simulink model "n2"  (R2013a)
settings: Solver=ode45  StartTime=0.0  StopTime=time  RelTol=1e-3
values from neighbouring files (symbols this model uses):
  noisePower = 1e3    (= 1000)    [proj.m]
undefined symbols (not defined in the file or in its folder): init, seed
libraries: neural x55, simulink x1
(part 2 of 3)

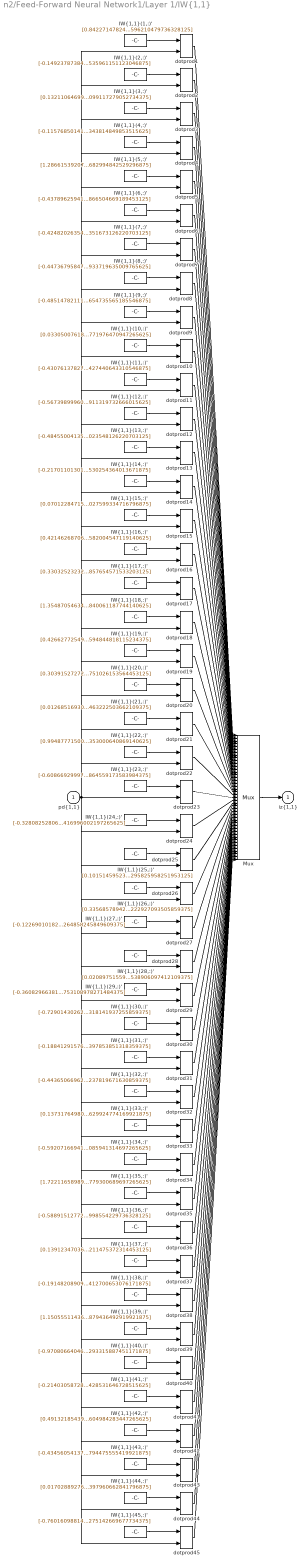
== system n2/Feed-Forward Neural Network1/Layer 1/IW{1,1} ==
  "pd{1,1}" : Inport  PortDimensions=6
      mask Display: e = 0.06;c1 = [120 230 180]/255;c2 = ([120 230 180]+0)/(256+128);c3 = ([120 230 180]+128)/(256+128);patch([0 1 1 0],[0 0 1 1],c1);patch([0 1 1 1-e 1-e 0+e],[0 0 1 1-e 0+e 0+e],c2);patch([0 0 1 1-e 0+e 0+e],[0 1 1 1-e 1-e 0+e],c3);plot([0 1 1 0 0],[0 0 1 1 0]);
  "IW{1,1}(1,:)'" : Constant  Value=[0.84227147824054549030137195586576126515865325927734375;0.06487427549836476126099427119697793386876583099365234375;0.16547979048669725354869797229184769093990325927734375;1.102066528263456302028089339728467166423797607421875;0.49259517334991442805147698891232721507549285888671875;-0.272176103875577724000578427876462228596210479736328125]
      mask Display: e = 0.06;c1 = [120 150 230]/255;c2 = ([120 150 230]+0)/383;c3 = ([120 150 230]+128)/383;patch([0 1 1 0],[0 0 1 1],c1);patch([0 1 1 1-e 1-e 0+e],[0 0 1 1-e 0+e 0+e],c2);patch([0 0 1 1-e 0+e 0+e],[0 1 1 1-e 1-e 0+e],c3);plot([0 1 1 0 0],[0 0 1 1 0]);disp('Weights');
  "IW{1,1}(10,:)'" : Constant  Value=[0.03305007618415702064229577672449522651731967926025390625;1.0170563445854501338772024610079824924468994140625;0.279931382798406624967668676617904566228389739990234375;0.426941937985293173962730861603631637990474700927734375;-1.5403738480250581677211130227078683674335479736328125;-0.91567469693016079190783784724771976470947265625]
      mask Display: e = 0.06;c1 = [120 150 230]/255;c2 = ([120 150 230]+0)/383;c3 = ([120 150 230]+128)/383;patch([0 1 1 0],[0 0 1 1],c1);patch([0 1 1 1-e 1-e 0+e],[0 0 1 1-e 0+e 0+e],c2);patch([0 0 1 1-e 0+e 0+e],[0 1 1 1-e 1-e 0+e],c3);plot([0 1 1 0 0],[0 0 1 1 0]);disp('Weights');
  "IW{1,1}(11,:)'" : Constant  Value=[-0.430761378274666040244511577839148230850696563720703125;3.4100337146199013460545756970532238483428955078125;-0.9436086074396683454068579521845094859600067138671875;-3.361420006301363283540695192641578614711761474609375;-3.569707650142730503972643418819643557071685791015625;-1.7836434418088156217407913572969846427440643310546875]
      mask Display: e = 0.06;c1 = [120 150 230]/255;c2 = ([120 150 230]+0)/383;c3 = ([120 150 230]+128)/383;patch([0 1 1 0],[0 0 1 1],c1);patch([0 1 1 1-e 1-e 0+e],[0 0 1 1-e 0+e 0+e],c2);patch([0 0 1 1-e 0+e 0+e],[0 1 1 1-e 1-e 0+e],c3);plot([0 1 1 0 0],[0 0 1 1 0]);disp('Weights');
  "IW{1,1}(12,:)'" : Constant  Value=[-0.5673989996097008603470612797536887228488922119140625;-1.41580995779519458466211290215142071247100830078125;1.9873570195839664886960918011027388274669647216796875;1.3572415823679129243117813530261628329753875732421875;1.0574804788789748943855784091283567249774932861328125;1.2123627937006260513186362004489637911319732666015625]
      mask Display: e = 0.06;c1 = [120 150 230]/255;c2 = ([120 150 230]+0)/383;c3 = ([120 150 230]+128)/383;patch([0 1 1 0],[0 0 1 1],c1);patch([0 1 1 1-e 1-e 0+e],[0 0 1 1-e 0+e 0+e],c2);patch([0 0 1 1-e 0+e 0+e],[0 1 1 1-e 1-e 0+e],c3);plot([0 1 1 0 0],[0 0 1 1 0]);disp('Weights');
  "IW{1,1}(13,:)'" : Constant  Value=[-0.48455004135934187647904991536051966249942779541015625;-0.7797168963881688785733103941311128437519073486328125;2.498924318770319619176234482438303530216217041015625;-1.7260272854251688112725560131366364657878875732421875;2.327445972270126173242488221148960292339324951171875;-0.05519446440998605762917605943584931083023548126220703125]
      mask Display: e = 0.06;c1 = [120 150 230]/255;c2 = ([120 150 230]+0)/383;c3 = ([120 150 230]+128)/383;patch([0 1 1 0],[0 0 1 1],c1);patch([0 1 1 1-e 1-e 0+e],[0 0 1 1-e 0+e 0+e],c2);patch([0 0 1 1-e 0+e 0+e],[0 1 1 1-e 1-e 0+e],c3);plot([0 1 1 0 0],[0 0 1 1 0]);disp('Weights');
  "IW{1,1}(14,:)'" : Constant  Value=[-0.21701101301024527945315867327735759317874908447265625;-0.08850209990518463631925527579369372688233852386474609375;1.269844430507898636051322682760655879974365234375;0.8399275689099445774132846054271794855594635009765625;-0.25354230062065064021936677818302996456623077392578125;-0.6468052937445747385680760999093763530254364013671875]
      mask Display: e = 0.06;c1 = [120 150 230]/255;c2 = ([120 150 230]+0)/383;c3 = ([120 150 230]+128)/383;patch([0 1 1 0],[0 0 1 1],c1);patch([0 1 1 1-e 1-e 0+e],[0 0 1 1-e 0+e 0+e],c2);patch([0 0 1 1-e 0+e 0+e],[0 1 1 1-e 1-e 0+e],c3);plot([0 1 1 0 0],[0 0 1 1 0]);disp('Weights');
  "IW{1,1}(15,:)'" : Constant  Value=[0.07012284715927970257798307329721865244209766387939453125;-0.426352730645800981346127400684054009616374969482421875;-0.462449000988150393798292725477949716150760650634765625;-1.848085497564675439008397006546147167682647705078125;-2.454998577026266115552743940497748553752899169921875;0.17757016677518588920747788506560027599334716796875]
      mask Display: e = 0.06;c1 = [120 150 230]/255;c2 = ([120 150 230]+0)/383;c3 = ([120 150 230]+128)/383;patch([0 1 1 0],[0 0 1 1],c1);patch([0 1 1 1-e 1-e 0+e],[0 0 1 1-e 0+e 0+e],c2);patch([0 0 1 1-e 0+e 0+e],[0 1 1 1-e 1-e 0+e],c3);plot([0 1 1 0 0],[0 0 1 1 0]);disp('Weights');
  "IW{1,1}(16,:)'" : Constant  Value=[0.4214626870610287401319737909943796694278717041015625;2.093231886567525013020940605201758444309234619140625;0.141001471649424725551824622016283683478832244873046875;0.50265377695913515676551241995184682309627532958984375;-0.44469249994842086071145104142487980425357818603515625;-2.61912069499532496053006980218924582004547119140625]
      mask Display: e = 0.06;c1 = [120 150 230]/255;c2 = ([120 150 230]+0)/383;c3 = ([120 150 230]+128)/383;patch([0 1 1 0],[0 0 1 1],c1);patch([0 1 1 1-e 1-e 0+e],[0 0 1 1-e 0+e 0+e],c2);patch([0 0 1 1-e 0+e 0+e],[0 1 1 1-e 1-e 0+e],c3);plot([0 1 1 0 0],[0 0 1 1 0]);disp('Weights');
  "IW{1,1}(17,:)'" : Constant  Value=[0.33032523232557242653939511001226492226123809814453125;4.676102860776463643333045183680951595306396484375;-0.55133479214566361026328422667575068771839141845703125;0.41738439187882947489782736738561652600765228271484375;-2.88390872632815131737515912391245365142822265625;0.559538075820381397562641723197884857654571533203125]
      mask Display: e = 0.06;c1 = [120 150 230]/255;c2 = ([120 150 230]+0)/383;c3 = ([120 150 230]+128)/383;patch([0 1 1 0],[0 0 1 1],c1);patch([0 1 1 1-e 1-e 0+e],[0 0 1 1-e 0+e 0+e],c2);patch([0 0 1 1-e 0+e 0+e],[0 1 1 1-e 1-e 0+e],c3);plot([0 1 1 0 0],[0 0 1 1 0]);disp('Weights');
  "IW{1,1}(18,:)'" : Constant  Value=[1.354870546341602643991564036696217954158782958984375;1.76135701700342650610764394514262676239013671875;0.2498693130782637938924750642399885691702365875244140625;0.018656499881086315018041688063021865673363208770751953125;-0.98870833590241102850626475628814660012722015380859375;-1.356004791091452776896630894043482840061187744140625]
      mask Display: e = 0.06;c1 = [120 150 230]/255;c2 = ([120 150 230]+0)/383;c3 = ([120 150 230]+128)/383;patch([0 1 1 0],[0 0 1 1],c1);patch([0 1 1 1-e 1-e 0+e],[0 0 1 1-e 0+e 0+e],c2);patch([0 0 1 1-e 0+e 0+e],[0 1 1 1-e 1-e 0+e],c3);plot([0 1 1 0 0],[0 0 1 1 0]);disp('Weights');
  "IW{1,1}(19,:)'" : Constant  Value=[0.42662772549766503349388813148834742605686187744140625;-4.7381878692336609759649945772252976894378662109375;-1.5030142946332050168933847089647315442562103271484375;-2.29340533164774029728505411185324192047119140625;-0.444288784337299291760103869819431565701961517333984375;1.437081857744058055459390743635594844818115234375]
      mask Display: e = 0.06;c1 = [120 150 230]/255;c2 = ([120 150 230]+0)/383;c3 = ([120 150 230]+128)/383;patch([0 1 1 0],[0 0 1 1],c1);patch([0 1 1 1-e 1-e 0+e],[0 0 1 1-e 0+e 0+e],c2);patch([0 0 1 1-e 0+e 0+e],[0 1 1 1-e 1-e 0+e],c3);plot([0 1 1 0 0],[0 0 1 1 0]);disp('Weights');
  "IW{1,1}(2,:)'" : Constant  Value=[-0.1492378738459924913950516156546655111014842987060546875;-0.58532240022470827245371083336067385971546173095703125;0.462664738325598789980830360946129076182842254638671875;1.91420588056120788422731493483297526836395263671875;-1.443266540980558954032630936126224696636199951171875;0.1477060064733095312572430657382938079535961151123046875]
      mask Display: e = 0.06;c1 = [120 150 230]/255;c2 = ([120 150 230]+0)/383;c3 = ([120 150 230]+128)/383;patch([0 1 1 0],[0 0 1 1],c1);patch([0 1 1 1-e 1-e 0+e],[0 0 1 1-e 0+e 0+e],c2);patch([0 0 1 1-e 0+e 0+e],[0 1 1 1-e 1-e 0+e],c3);plot([0 1 1 0 0],[0 0 1 1 0]);disp('Weights');
  "IW{1,1}(20,:)'" : Constant  Value=[0.30391527272730389785948545977589674293994903564453125;-0.444187486126631114746743378418614156544208526611328125;-0.022000359677070625841199813521598116494715213775634765625;-0.5972509067636926349820214454666711390018463134765625;2.6133128367743925224431222886778414249420166015625;2.22748035673238309328780815121717751026153564453125]
      mask Display: e = 0.06;c1 = [120 150 230]/255;c2 = ([120 150 230]+0)/383;c3 = ([120 150 230]+128)/383;patch([0 1 1 0],[0 0 1 1],c1);patch([0 1 1 1-e 1-e 0+e],[0 0 1 1-e 0+e 0+e],c2);patch([0 0 1 1-e 0+e 0+e],[0 1 1 1-e 1-e 0+e],c3);plot([0 1 1 0 0],[0 0 1 1 0]);disp('Weights');
  "IW{1,1}(21,:)'" : Constant  Value=[0.01268516930794892638711957033592625521123409271240234375;4.59450107657331141552958797547034919261932373046875;-0.93306119762650896465316918693133629858493804931640625;-1.6092357280682261233550889301113784313201904296875;-3.214514491239682580925318688969127833843231201171875;-0.6781370341470525087146370424306951463222503662109375]
      mask Display: e = 0.06;c1 = [120 150 230]/255;c2 = ([120 150 230]+0)/383;c3 = ([120 150 230]+128)/383;patch([0 1 1 0],[0 0 1 1],c1);patch([0 1 1 1-e 1-e 0+e],[0 0 1 1-e 0+e 0+e],c2);patch([0 0 1 1-e 0+e 0+e],[0 1 1 1-e 1-e 0+e],c3);plot([0 1 1 0 0],[0 0 1 1 0]);disp('Weights');
  "IW{1,1}(22,:)'" : Constant  Value=[0.994877715005721530161508781020529568195343017578125;-2.5852327063540183615941714379005134105682373046875;-0.4537861220633285785908128673327155411243438720703125;0.74245142888689319438100255865720100700855255126953125;-1.833503204946538289732416160404682159423828125;15.454823990822948331924635567702353000640869140625]
      mask Display: e = 0.06;c1 = [120 150 230]/255;c2 = ([120 150 230]+0)/383;c3 = ([120 150 230]+128)/383;patch([0 1 1 0],[0 0 1 1],c1);patch([0 1 1 1-e 1-e 0+e],[0 0 1 1-e 0+e 0+e],c2);patch([0 0 1 1-e 0+e 0+e],[0 1 1 1-e 1-e 0+e],c3);plot([0 1 1 0 0],[0 0 1 1 0]);disp('Weights');
  "IW{1,1}(23,:)'" : Constant  Value=[-0.60866929997868346458034238821710459887981414794921875;-0.97057598832021951817949911855976097285747528076171875;-1.41630044446994940443573796073906123638153076171875;1.6145332171968866941114129076595418155193328857421875;1.9343143141262479911546279254253022372722625732421875;3.68592187714530350461927810101769864559173583984375]
      mask Display: e = 0.06;c1 = [120 150 230]/255;c2 = ([120 150 230]+0)/383;c3 = ([120 150 230]+128)/383;patch([0 1 1 0],[0 0 1 1],c1);patch([0 1 1 1-e 1-e 0+e],[0 0 1 1-e 0+e 0+e],c2);patch([0 0 1 1-e 0+e 0+e],[0 1 1 1-e 1-e 0+e],c3);plot([0 1 1 0 0],[0 0 1 1 0]);disp('Weights');
  "IW{1,1}(24,:)'" : Constant  Value=[-0.32808252806051185768154709876398555934429168701171875;-3.42123638500376170412664578179828822612762451171875;-0.904267633019632643964769158628769218921661376953125;0.74638609472593231419779158386518247425556182861328125;1.925961651847787781122178785153664648532867431640625;-0.1414651721659340444237074052580283023416996002197265625]
      mask Display: e = 0.06;c1 = [120 150 230]/255;c2 = ([120 150 230]+0)/383;c3 = ([120 150 230]+128)/383;patch([0 1 1 0],[0 0 1 1],c1);patch([0 1 1 1-e 1-e 0+e],[0 0 1 1-e 0+e 0+e],c2);patch([0 0 1 1-e 0+e 0+e],[0 1 1 1-e 1-e 0+e],c3);plot([0 1 1 0 0],[0 0 1 1 0]);disp('Weights');
  "IW{1,1}(25,:)'" : Constant  Value=[0.1015145952320345157371406230595312081277370452880859375;-0.332514223086164684151100345843588002026081085205078125;2.281582187239048042926015114062465727329254150390625;0.83332205829804639751756667465087957680225372314453125;-1.74625792582558414522964085335843265056610107421875;0.9113021358531601112673570241895504295825958251953125]
      mask Display: e = 0.06;c1 = [120 150 230]/255;c2 = ([120 150 230]+0)/383;c3 = ([120 150 230]+128)/383;patch([0 1 1 0],[0 0 1 1],c1);patch([0 1 1 1-e 1-e 0+e],[0 0 1 1-e 0+e 0+e],c2);patch([0 0 1 1-e 0+e 0+e],[0 1 1 1-e 1-e 0+e],c3);plot([0 1 1 0 0],[0 0 1 1 0]);disp('Weights');
  "IW{1,1}(26,:)'" : Constant  Value=[0.33568578942289628574968674001866020262241363525390625;2.3543740308923606363578073796816170215606689453125;1.351961238632386486102632261463440954685211181640625;1.7606296753255026299456176275270991027355194091796875;-0.41700357843252511269582782915676943957805633544921875;1.0395595474903343014005940858623944222927093505859375]
      mask Display: e = 0.06;c1 = [120 150 230]/255;c2 = ([120 150 230]+0)/383;c3 = ([120 150 230]+128)/383;patch([0 1 1 0],[0 0 1 1],c1);patch([0 1 1 1-e 1-e 0+e],[0 0 1 1-e 0+e 0+e],c2);patch([0 0 1 1-e 0+e 0+e],[0 1 1 1-e 1-e 0+e],c3);plot([0 1 1 0 0],[0 0 1 1 0]);disp('Weights');
  "IW{1,1}(27,:)'" : Constant  Value=[-0.122690101827504116638323239385499618947505950927734375;-4.38180574480759066346990948659367859363555908203125;-0.93975792619900133662014241053839214146137237548828125;-1.477176900329489672714089465443976223468780517578125;-0.1684666325636204053939337654810515232384204864501953125;0.372092735345911085342862634206539951264858245849609375]
      mask Display: e = 0.06;c1 = [120 150 230]/255;c2 = ([120 150 230]+0)/383;c3 = ([120 150 230]+128)/383;patch([0 1 1 0],[0 0 1 1],c1);patch([0 1 1 1-e 1-e 0+e],[0 0 1 1-e 0+e 0+e],c2);patch([0 0 1 1-e 0+e 0+e],[0 1 1 1-e 1-e 0+e],c3);plot([0 1 1 0 0],[0 0 1 1 0]);disp('Weights');
  "IW{1,1}(28,:)'" : Constant  Value=[0.0208975155955787202100015775840802234597504138946533203125;1.251660217050768242330605062306858599185943603515625;1.1691366816001658168744370414060540497303009033203125;2.7047155750761060488684961455874145030975341796875;2.570977437632034234837874464574269950389862060546875;-0.1415574810387700832592372535145841538906097412109375]
      mask Display: e = 0.06;c1 = [120 150 230]/255;c2 = ([120 150 230]+0)/383;c3 = ([120 150 230]+128)/383;patch([0 1 1 0],[0 0 1 1],c1);patch([0 1 1 1-e 1-e 0+e],[0 0 1 1-e 0+e 0+e],c2);patch([0 0 1 1-e 0+e 0+e],[0 1 1 1-e 1-e 0+e],c3);plot([0 1 1 0 0],[0 0 1 1 0]);disp('Weights');
  "IW{1,1}(29,:)'" : Constant  Value=[-0.360829663811210121782124815581482835114002227783203125;-0.88319440128383386312549419017159380018711090087890625;3.3498526307737837015565673937089741230010986328125;1.233805697106404419827185847680084407329559326171875;-0.10885207267648533413506584111019037663936614990234375;-0.7884649843305184813146979649900458753108978271484375]
      mask Display: e = 0.06;c1 = [120 150 230]/255;c2 = ([120 150 230]+0)/383;c3 = ([120 150 230]+128)/383;patch([0 1 1 0],[0 0 1 1],c1);patch([0 1 1 1-e 1-e 0+e],[0 0 1 1-e 0+e 0+e],c2);patch([0 0 1 1-e 0+e 0+e],[0 1 1 1-e 1-e 0+e],c3);plot([0 1 1 0 0],[0 0 1 1 0]);disp('Weights');
  "IW{1,1}(3,:)'" : Constant  Value=[0.1321106469977538500071290172854787670075893402099609375;-0.397375057727925751205333426696597598493099212646484375;-0.042944704991947350858350063163015875034034252166748046875;1.599760712104874027517098511452786624431610107421875;0.2558827644516330490631617067265324294567108154296875;0.4060595418232446629502874202444218099117279052734375]
      mask Display: e = 0.06;c1 = [120 150 230]/255;c2 = ([120 150 230]+0)/383;c3 = ([120 150 230]+128)/383;patch([0 1 1 0],[0 0 1 1],c1);patch([0 1 1 1-e 1-e 0+e],[0 0 1 1-e 0+e 0+e],c2);patch([0 0 1 1-e 0+e 0+e],[0 1 1 1-e 1-e 0+e],c3);plot([0 1 1 0 0],[0 0 1 1 0]);disp('Weights');
  "IW{1,1}(30,:)'" : Constant  Value=[-0.7290143026208630860907078385935164988040924072265625;-1.506358840224149897579764001420699059963226318359375;-0.47719700980047574656595088526955805718898773193359375;0.3448008435778924241077447732095606625080108642578125;0.06901407753184805871082829753504483960568904876708984375;2.197857444031098506087573696277104318141937255859375]
      mask Display: e = 0.06;c1 = [120 150 230]/255;c2 = ([120 150 230]+0)/383;c3 = ([120 150 230]+128)/383;patch([0 1 1 0],[0 0 1 1],c1);patch([0 1 1 1-e 1-e 0+e],[0 0 1 1-e 0+e 0+e],c2);patch([0 0 1 1-e 0+e 0+e],[0 1 1 1-e 1-e 0+e],c3);plot([0 1 1 0 0],[0 0 1 1 0]);disp('Weights');
  "IW{1,1}(31,:)'" : Constant  Value=[-0.18841291576789931383473231107927858829498291015625;-1.883810688531983856819351785816252231597900390625;-1.528012023680080933019098665681667625904083251953125;-2.989909602536509058978708708309568464756011962890625;-1.5647943251507172579550797308911569416522979736328125;-0.47964740637355018915144455604604445397853851318359375]
      mask Display: e = 0.06;c1 = [120 150 230]/255;c2 = ([120 150 230]+0)/383;c3 = ([120 150 230]+128)/383;patch([0 1 1 0],[0 0 1 1],c1);patch([0 1 1 1-e 1-e 0+e],[0 0 1 1-e 0+e 0+e],c2);patch([0 0 1 1-e 0+e 0+e],[0 1 1 1-e 1-e 0+e],c3);plot([0 1 1 0 0],[0 0 1 1 0]);disp('Weights');
  "IW{1,1}(32,:)'" : Constant  Value=[-0.443650669627721538912368259843788109719753265380859375;-1.4009311657658527483505395139218308031558990478515625;-2.2726150371821116635828730068169534206390380859375;-0.2245478230346547865448059155824012123048305511474609375;-0.1355220260937668175227344136146712116897106170654296875;1.084261365339057814338730167946778237819671630859375]
      mask Display: e = 0.06;c1 = [120 150 230]/255;c2 = ([120 150 230]+0)/383;c3 = ([120 150 230]+128)/383;patch([0 1 1 0],[0 0 1 1],c1);patch([0 1 1 1-e 1-e 0+e],[0 0 1 1-e 0+e 0+e],c2);patch([0 0 1 1-e 0+e 0+e],[0 1 1 1-e 1-e 0+e],c3);plot([0 1 1 0 0],[0 0 1 1 0]);disp('Weights');
  "IW{1,1}(33,:)'" : Constant  Value=[0.137317649806484365360148558465880341827869415283203125;-0.55945470154716614441525734946480952203273773193359375;3.618543150025871124597642847220413386821746826171875;3.33383798934054720319863918120972812175750732421875;-0.822871208637542483899096623645164072513580322265625;1.5973819108851479153798891275073401629924774169921875]
      mask Display: e = 0.06;c1 = [120 150 230]/255;c2 = ([120 150 230]+0)/383;c3 = ([120 150 230]+128)/383;patch([0 1 1 0],[0 0 1 1],c1);patch([0 1 1 1-e 1-e 0+e],[0 0 1 1-e 0+e 0+e],c2);patch([0 0 1 1-e 0+e 0+e],[0 1 1 1-e 1-e 0+e],c3);plot([0 1 1 0 0],[0 0 1 1 0]);disp('Weights');
  "IW{1,1}(34,:)'" : Constant  Value=[-0.592071669418371637760856174281798303127288818359375;-0.83421267712764202162389892691862769424915313720703125;0.86348993686630171051632487433380447328090667724609375;2.150819845230817151104929507710039615631103515625;2.262924582499760361997687141411006450653076171875;-0.0255007571660771405197554173582830117084085941314697265625]
      mask Display: e = 0.06;c1 = [120 150 230]/255;c2 = ([120 150 230]+0)/383;c3 = ([120 150 230]+128)/383;patch([0 1 1 0],[0 0 1 1],c1);patch([0 1 1 1-e 1-e 0+e],[0 0 1 1-e 0+e 0+e],c2);patch([0 0 1 1-e 0+e 0+e],[0 1 1 1-e 1-e 0+e],c3);plot([0 1 1 0 0],[0 0 1 1 0]);disp('Weights');
  "IW{1,1}(35,:)'" : Constant  Value=[1.7221165898979722275186077240505255758762359619140625;3.29144936960714229456925750127993524074554443359375;-0.70751409013431487693424060125835239887237548828125;-1.0795418691169966773912847202154807746410369873046875;-1.105857120792361314443041919730603694915771484375;-1.502964798220688180663273669779300689697265625]
      mask Display: e = 0.06;c1 = [120 150 230]/255;c2 = ([120 150 230]+0)/383;c3 = ([120 150 230]+128)/383;patch([0 1 1 0],[0 0 1 1],c1);patch([0 1 1 1-e 1-e 0+e],[0 0 1 1-e 0+e 0+e],c2);patch([0 0 1 1-e 0+e 0+e],[0 1 1 1-e 1-e 0+e],c3);plot([0 1 1 0 0],[0 0 1 1 0]);disp('Weights');
  "IW{1,1}(36,:)'" : Constant  Value=[-0.58891512772877174786145815232885070145130157470703125;-4.9511689644958014611120233894325792789459228515625;-2.23201641639018699692087466246448457241058349609375;1.0115433068301593610982536119990982115268707275390625;2.87365060958359297416109257028438150882720947265625;-0.22953357547706787489261159862508065998554229736328125]
      mask Display: e = 0.06;c1 = [120 150 230]/255;c2 = ([120 150 230]+0)/383;c3 = ([120 150 230]+128)/383;patch([0 1 1 0],[0 0 1 1],c1);patch([0 1 1 1-e 1-e 0+e],[0 0 1 1-e 0+e 0+e],c2);patch([0 0 1 1-e 0+e 0+e],[0 1 1 1-e 1-e 0+e],c3);plot([0 1 1 0 0],[0 0 1 1 0]);disp('Weights');
  "IW{1,1}(37,:)'" : Constant  Value=[0.139123470369716617511812728480435907840728759765625;-1.289834396248152881270243597100488841533660888671875;0.2722104703413099624498272532946430146694183349609375;0.261716197281477269687144371346221305429935455322265625;-0.797707282571357811917778235510922968387603759765625;0.57652892523213428166428684562561102211475372314453125]
      mask Display: e = 0.06;c1 = [120 150 230]/255;c2 = ([120 150 230]+0)/383;c3 = ([120 150 230]+128)/383;patch([0 1 1 0],[0 0 1 1],c1);patch([0 1 1 1-e 1-e 0+e],[0 0 1 1-e 0+e 0+e],c2);patch([0 0 1 1-e 0+e 0+e],[0 1 1 1-e 1-e 0+e],c3);plot([0 1 1 0 0],[0 0 1 1 0]);disp('Weights');
  "IW{1,1}(38,:)'" : Constant  Value=[-0.1914820890937098674111638274553115479648113250732421875;7.38545949292279413356254735845141112804412841796875;-0.487500818685457637524649499027873389422893524169921875;0.1196565559715188076239655856625176966190338134765625;0.1946593969480634456203915760852396488189697265625;0.347467836883841030282127348982612602412700653076171875]
      mask Display: e = 0.06;c1 = [120 150 230]/255;c2 = ([120 150 230]+0)/383;c3 = ([120 150 230]+128)/383;patch([0 1 1 0],[0 0 1 1],c1);patch([0 1 1 1-e 1-e 0+e],[0 0 1 1-e 0+e 0+e],c2);patch([0 0 1 1-e 0+e 0+e],[0 1 1 1-e 1-e 0+e],c3);plot([0 1 1 0 0],[0 0 1 1 0]);disp('Weights');
  "IW{1,1}(39,:)'" : Constant  Value=[1.1505551143686323367631985092884860932826995849609375;0.670927704314908002203310388722456991672515869140625;-0.4107825063660275333177196444012224674224853515625;0.34580825776955259609479753635241650044918060302734375;0.273933720244461442749894786174991168081760406494140625;0.10240294396416320388265575047626043669879436492919921875]
      mask Display: e = 0.06;c1 = [120 150 230]/255;c2 = ([120 150 230]+0)/383;c3 = ([120 150 230]+128)/383;patch([0 1 1 0],[0 0 1 1],c1);patch([0 1 1 1-e 1-e 0+e],[0 0 1 1-e 0+e 0+e],c2);patch([0 0 1 1-e 0+e 0+e],[0 1 1 1-e 1-e 0+e],c3);plot([0 1 1 0 0],[0 0 1 1 0]);disp('Weights');
  "IW{1,1}(4,:)'" : Constant  Value=[-0.11576850141052537346286754882385139353573322296142578125;-4.54558036892190120425993882236070930957794189453125;-0.092313141273975052314426648081280291080474853515625;0.12126186077174672117706677454407326877117156982421875;0.1615396998211687529245494943097583018243312835693359375;0.10394610992355980683132798958467901684343814849853515625]
      mask Display: e = 0.06;c1 = [120 150 230]/255;c2 = ([120 150 230]+0)/383;c3 = ([120 150 230]+128)/383;patch([0 1 1 0],[0 0 1 1],c1);patch([0 1 1 1-e 1-e 0+e],[0 0 1 1-e 0+e 0+e],c2);patch([0 0 1 1-e 0+e 0+e],[0 1 1 1-e 1-e 0+e],c3);plot([0 1 1 0 0],[0 0 1 1 0]);disp('Weights');
  "IW{1,1}(40,:)'" : Constant  Value=[-0.9708066404631108259337679555756039917469024658203125;-0.72668604922306612170501693981350399553775787353515625;0.891458005586482915560964102041907608509063720703125;1.253717701823703567498569100280292332172393798828125;0.8892087248039166613722272813902236521244049072265625;0.1584588009797140983891949872486293315887451171875]
      mask Display: e = 0.06;c1 = [120 150 230]/255;c2 = ([120 150 230]+0)/383;c3 = ([120 150 230]+128)/383;patch([0 1 1 0],[0 0 1 1],c1);patch([0 1 1 1-e 1-e 0+e],[0 0 1 1-e 0+e 0+e],c2);patch([0 0 1 1-e 0+e 0+e],[0 1 1 1-e 1-e 0+e],c3);plot([0 1 1 0 0],[0 0 1 1 0]);disp('Weights');
  "IW{1,1}(41,:)'" : Constant  Value=[-0.214030587285944040587537529063411056995391845703125;0.81855538866011212650874995233607478439807891845703125;0.5267935584121830050463586303521879017353057861328125;-0.369976614021223060291276851785369217395782470703125;0.75418730631755803717197750302148051559925079345703125;0.62987453426894701724592096070409752428531646728515625]
      mask Display: e = 0.06;c1 = [120 150 230]/255;c2 = ([120 150 230]+0)/383;c3 = ([120 150 230]+128)/383;patch([0 1 1 0],[0 0 1 1],c1);patch([0 1 1 1-e 1-e 0+e],[0 0 1 1-e 0+e 0+e],c2);patch([0 0 1 1-e 0+e 0+e],[0 1 1 1-e 1-e 0+e],c3);plot([0 1 1 0 0],[0 0 1 1 0]);disp('Weights');
  "IW{1,1}(42,:)'" : Constant  Value=[0.491321854398087454196542012141435407102108001708984375;-0.6243604795551085384630596308852545917034149169921875;-0.8073042670592747160895896740839816629886627197265625;-0.4604107257932936736466444926918484270572662353515625;-0.2307547176901788843483842583736986853182315826416015625;-0.11031798080602052414267433277927921153604984283447265625]
      mask Display: e = 0.06;c1 = [120 150 230]/255;c2 = ([120 150 230]+0)/383;c3 = ([120 150 230]+128)/383;patch([0 1 1 0],[0 0 1 1],c1);patch([0 1 1 1-e 1-e 0+e],[0 0 1 1-e 0+e 0+e],c2);patch([0 0 1 1-e 0+e 0+e],[0 1 1 1-e 1-e 0+e],c3);plot([0 1 1 0 0],[0 0 1 1 0]);disp('Weights');
  "IW{1,1}(43,:)'" : Constant  Value=[-0.434560541377054743161778560534003190696239471435546875;-0.7195817968029818434416711170342750847339630126953125;2.719625083265178044911181132192723453044891357421875;-0.9651400988834157868012653125333599746227264404296875;-1.8899754067195717599503268502303399145603179931640625;0.2358315585990613250100267350717331282794475555419921875]
      mask Display: e = 0.06;c1 = [120 150 230]/255;c2 = ([120 150 230]+0)/383;c3 = ([120 150 230]+128)/383;patch([0 1 1 0],[0 0 1 1],c1);patch([0 1 1 1-e 1-e 0+e],[0 0 1 1-e 0+e 0+e],c2);patch([0 0 1 1-e 0+e 0+e],[0 1 1 1-e 1-e 0+e],c3);plot([0 1 1 0 0],[0 0 1 1 0]);disp('Weights');
  "IW{1,1}(44,:)'" : Constant  Value=[0.0170288927643164507419459852144427713938057422637939453125;-1.096271515043029776137473163544200360774993896484375;-0.65716506950018771515686921702581457793712615966796875;-2.615029860688120155742808492504991590976715087890625;0.185285386266270502009234633078449405729770660400390625;0.6822539905081999034308637419599108397960662841796875]
      mask Display: e = 0.06;c1 = [120 150 230]/255;c2 = ([120 150 230]+0)/383;c3 = ([120 150 230]+128)/383;patch([0 1 1 0],[0 0 1 1],c1);patch([0 1 1 1-e 1-e 0+e],[0 0 1 1-e 0+e 0+e],c2);patch([0 0 1 1-e 0+e 0+e],[0 1 1 1-e 1-e 0+e],c3);plot([0 1 1 0 0],[0 0 1 1 0]);disp('Weights');
  "IW{1,1}(45,:)'" : Constant  Value=[-0.76016098814205346201333668432198464870452880859375;0.45662035591078098395456663638469763100147247314453125;-0.69560184134009650502861177301383577287197113037109375;0.05786432331366657411120257847869652323424816131591796875;-0.415050499588511423443293324453406967222690582275390625;0.85467177567879326627320324405445717275142669677734375]
      mask Display: e = 0.06;c1 = [120 150 230]/255;c2 = ([120 150 230]+0)/383;c3 = ([120 150 230]+128)/383;patch([0 1 1 0],[0 0 1 1],c1);patch([0 1 1 1-e 1-e 0+e],[0 0 1 1-e 0+e 0+e],c2);patch([0 0 1 1-e 0+e 0+e],[0 1 1 1-e 1-e 0+e],c3);plot([0 1 1 0 0],[0 0 1 1 0]);disp('Weights');
  "IW{1,1}(5,:)'" : Constant  Value=[1.286615392073253705262914081686176359653472900390625;-0.63236160984545997099104397420887835323810577392578125;1.0393417445908534890719465693109668791294097900390625;-1.0017921343315656645955868953024037182331085205078125;1.2961703714111709739853495193528942763805389404296875;0.69475220751266686392000337946228682994842529296875]
      mask Display: e = 0.06;c1 = [120 150 230]/255;c2 = ([120 150 230]+0)/383;c3 = ([120 150 230]+128)/383;patch([0 1 1 0],[0 0 1 1],c1);patch([0 1 1 1-e 1-e 0+e],[0 0 1 1-e 0+e 0+e],c2);patch([0 0 1 1-e 0+e 0+e],[0 1 1 1-e 1-e 0+e],c3);plot([0 1 1 0 0],[0 0 1 1 0]);disp('Weights');
  "IW{1,1}(6,:)'" : Constant  Value=[-0.437896259415833932759909430387779138982295989990234375;-0.055678103401010682615979163756492198444902896881103515625;0.86210316000251119294972568241064436733722686767578125;-1.2571776590128809214519378656405024230480194091796875;1.91653411562610020979491309844888746738433837890625;-1.175738488899714440094612655229866504669189453125]
      mask Display: e = 0.06;c1 = [120 150 230]/255;c2 = ([120 150 230]+0)/383;c3 = ([120 150 230]+128)/383;patch([0 1 1 0],[0 0 1 1],c1);patch([0 1 1 1-e 1-e 0+e],[0 0 1 1-e 0+e 0+e],c2);patch([0 0 1 1-e 0+e 0+e],[0 1 1 1-e 1-e 0+e],c3);plot([0 1 1 0 0],[0 0 1 1 0]);disp('Weights');
  "IW{1,1}(7,:)'" : Constant  Value=[-0.424820263545935716820167726837098598480224609375;0.0921595173958678903769481394192553125321865081787109375;1.5124409214377152466113329865038394927978515625;2.25606477612466083115805304259993135929107666015625;0.8804375291908701495202649311977438628673553466796875;-0.493414946284316979774331457520020194351673126220703125]
      mask Display: e = 0.06;c1 = [120 150 230]/255;c2 = ([120 150 230]+0)/383;c3 = ([120 150 230]+128)/383;patch([0 1 1 0],[0 0 1 1],c1);patch([0 1 1 1-e 1-e 0+e],[0 0 1 1-e 0+e 0+e],c2);patch([0 0 1 1-e 0+e 0+e],[0 1 1 1-e 1-e 0+e],c3);plot([0 1 1 0 0],[0 0 1 1 0]);disp('Weights');
  "IW{1,1}(8,:)'" : Constant  Value=[-0.447367958470151594330133093535550870001316070556640625;-0.57162951790862592815756215713918209075927734375;1.068904226705254867368921622983179986476898193359375;-0.36300666989660701489128769026137888431549072265625;0.0233603725425067278165247586230179877020418643951416015625;0.371345504439733409274282394108013249933719635009765625]
      mask Display: e = 0.06;c1 = [120 150 230]/255;c2 = ([120 150 230]+0)/383;c3 = ([120 150 230]+128)/383;patch([0 1 1 0],[0 0 1 1],c1);patch([0 1 1 1-e 1-e 0+e],[0 0 1 1-e 0+e 0+e],c2);patch([0 0 1 1-e 0+e 0+e],[0 1 1 1-e 1-e 0+e],c3);plot([0 1 1 0 0],[0 0 1 1 0]);disp('Weights');
  "IW{1,1}(9,:)'" : Constant  Value=[-0.485147821115319788365383146810927428305149078369140625;-1.5183877630525406399186749695218168199062347412109375;-3.14651794382773264402430868358351290225982666015625;-1.27616307751824020755293531692586839199066162109375;0.7526174427896663576831315367599017918109893798828125;1.599932614473981384861644983175210654735565185546875]
      mask Display: e = 0.06;c1 = [120 150 230]/255;c2 = ([120 150 230]+0)/383;c3 = ([120 150 230]+128)/383;patch([0 1 1 0],[0 0 1 1],c1);patch([0 1 1 1-e 1-e 0+e],[0 0 1 1-e 0+e 0+e],c2);patch([0 0 1 1-e 0+e 0+e],[0 1 1 1-e 1-e 0+e],c3);plot([0 1 1 0 0],[0 0 1 1 0]);disp('Weights');
  Mux : Mux  Inputs=45
      mask Display: e = 0.06;c1 = [120 150 230]/255;c2 = ([120 150 230]+0)/383;c3 = ([120 150 230]+128)/383;patch([0 1 1 0],[0 0 1 1],c1);patch([0 1 1 1-e 1-e 0+e],[0 0 1 1-e 0+e 0+e],c2);patch([0 0 1 1-e 0+e 0+e],[0 1 1 1-e 1-e 0+e],c3);plot([0 1 1 0 0],[0 0 1 1 0]);disp('Mux');
  dotprod{1..45} (45 alike) : neural/Weight Functions/dotprod
  "iz{1,1}" : Outport
      mask Display: e = 0.06;c1 = [120 230 180]/255;c2 = ([120 230 180]+0)/(256+128);c3 = ([120 230 180]+128)/(256+128);patch([0 1 1 0],[0 0 1 1],c1);patch([0 1 1 1-e 1-e 0+e],[0 0 1 1-e 0+e 0+e],c2);patch([0 0 1 1-e 0+e 0+e],[0 1 1 1-e 1-e 0+e],c3);plot([0 1 1 0 0],[0 0 1 1 0]);
  wires:
  "IW{1,1}(1,:)'"/1 -> dotprod1/1
  "pd{1,1}"/1 -> dotprod1/2, dotprod2/2, dotprod3/2, dotprod4/2, dotprod5/2, dotprod6/2, dotprod7/2, dotprod8/2, dotprod9/2, dotprod10/2, dotprod11/2, dotprod12/2, dotprod13/2, dotprod14/2, dotprod15/2, dotprod16/2, dotprod17/2, dotprod18/2, dotprod19/2, dotprod20/2, dotprod21/2, dotprod22/2, dotprod23/2, dotprod24/2, dotprod25/2, dotprod26/2, dotprod27/2, dotprod28/2, dotprod29/2, dotprod30/2, dotprod31/2, dotprod32/2, dotprod33/2, dotprod34/2, dotprod35/2, dotprod36/2, dotprod37/2, dotprod38/2, dotprod39/2, dotprod40/2, dotprod41/2, dotprod42/2, dotprod43/2, dotprod44/2, dotprod45/2
  dotprod1/1 -> Mux/1
  "IW{1,1}(2,:)'"/1 -> dotprod2/1
  dotprod2/1 -> Mux/2
  "IW{1,1}(3,:)'"/1 -> dotprod3/1
  dotprod3/1 -> Mux/3
  "IW{1,1}(4,:)'"/1 -> dotprod4/1
  dotprod4/1 -> Mux/4
  "IW{1,1}(5,:)'"/1 -> dotprod5/1
  dotprod5/1 -> Mux/5
  "IW{1,1}(6,:)'"/1 -> dotprod6/1
  dotprod6/1 -> Mux/6
  "IW{1,1}(7,:)'"/1 -> dotprod7/1
  dotprod7/1 -> Mux/7
  "IW{1,1}(8,:)'"/1 -> dotprod8/1
  dotprod8/1 -> Mux/8
  "IW{1,1}(9,:)'"/1 -> dotprod9/1
  dotprod9/1 -> Mux/9
  "IW{1,1}(10,:)'"/1 -> dotprod10/1
  dotprod10/1 -> Mux/10
  "IW{1,1}(11,:)'"/1 -> dotprod11/1
  dotprod11/1 -> Mux/11
  "IW{1,1}(12,:)'"/1 -> dotprod12/1
  dotprod12/1 -> Mux/12
  "IW{1,1}(13,:)'"/1 -> dotprod13/1
  dotprod13/1 -> Mux/13
  "IW{1,1}(14,:)'"/1 -> dotprod14/1
  dotprod14/1 -> Mux/14
  "IW{1,1}(15,:)'"/1 -> dotprod15/1
  dotprod15/1 -> Mux/15
  "IW{1,1}(16,:)'"/1 -> dotprod16/1
  dotprod16/1 -> Mux/16
  "IW{1,1}(17,:)'"/1 -> dotprod17/1
  dotprod17/1 -> Mux/17
  "IW{1,1}(18,:)'"/1 -> dotprod18/1
  dotprod18/1 -> Mux/18
  "IW{1,1}(19,:)'"/1 -> dotprod19/1
  dotprod19/1 -> Mux/19
  "IW{1,1}(20,:)'"/1 -> dotprod20/1
  dotprod20/1 -> Mux/20
  "IW{1,1}(21,:)'"/1 -> dotprod21/1
  dotprod21/1 -> Mux/21
  "IW{1,1}(22,:)'"/1 -> dotprod22/1
  dotprod22/1 -> Mux/22
  "IW{1,1}(23,:)'"/1 -> dotprod23/1
  dotprod23/1 -> Mux/23
  "IW{1,1}(24,:)'"/1 -> dotprod24/1
  dotprod24/1 -> Mux/24
  "IW{1,1}(25,:)'"/1 -> dotprod25/1
  dotprod25/1 -> Mux/25
  "IW{1,1}(26,:)'"/1 -> dotprod26/1
  dotprod26/1 -> Mux/26
  "IW{1,1}(27,:)'"/1 -> dotprod27/1
  dotprod27/1 -> Mux/27
  "IW{1,1}(28,:)'"/1 -> dotprod28/1
  dotprod28/1 -> Mux/28
  "IW{1,1}(29,:)'"/1 -> dotprod29/1
  dotprod29/1 -> Mux/29
  "IW{1,1}(30,:)'"/1 -> dotprod30/1
  dotprod30/1 -> Mux/30
  "IW{1,1}(31,:)'"/1 -> dotprod31/1
  dotprod31/1 -> Mux/31
  "IW{1,1}(32,:)'"/1 -> dotprod32/1
  dotprod32/1 -> Mux/32
  "IW{1,1}(33,:)'"/1 -> dotprod33/1
  dotprod33/1 -> Mux/33
  "IW{1,1}(34,:)'"/1 -> dotprod34/1
  dotprod34/1 -> Mux/34
  "IW{1,1}(35,:)'"/1 -> dotprod35/1
  dotprod35/1 -> Mux/35
  "IW{1,1}(36,:)'"/1 -> dotprod36/1
  dotprod36/1 -> Mux/36
  "IW{1,1}(37,:)'"/1 -> dotprod37/1
  dotprod37/1 -> Mux/37
  "IW{1,1}(38,:)'"/1 -> dotprod38/1
  dotprod38/1 -> Mux/38
  "IW{1,1}(39,:)'"/1 -> dotprod39/1
  dotprod39/1 -> Mux/39
  "IW{1,1}(40,:)'"/1 -> dotprod40/1
  dotprod40/1 -> Mux/40
  "IW{1,1}(41,:)'"/1 -> dotprod41/1
  dotprod41/1 -> Mux/41
  "IW{1,1}(42,:)'"/1 -> dotprod42/1
  dotprod42/1 -> Mux/42
  "IW{1,1}(43,:)'"/1 -> dotprod43/1
  dotprod43/1 -> Mux/43
  "IW{1,1}(44,:)'"/1 -> dotprod44/1
  dotprod44/1 -> Mux/44
  "IW{1,1}(45,:)'"/1 -> dotprod45/1
  dotprod45/1 -> Mux/45
  Mux/1 -> "iz{1,1}"/1

== system n2/Feed-Forward Neural Network1/Layer 2/Delays 1 ==
  "p{2}" : Inport  PortDimensions=45
      mask Display: e = 0.06;c1 = [120 230 180]/255;c2 = ([120 230 180]+0)/(256+128);c3 = ([120 230 180]+128)/(256+128);patch([0 1 1 0],[0 0 1 1],c1);patch([0 1 1 1-e 1-e 0+e],[0 0 1 1-e 0+e 0+e],c2);patch([0 0 1 1-e 0+e 0+e],[0 1 1 1-e 1-e 0+e],c3);plot([0 1 1 0 0],[0 0 1 1 0]);
  mux : Mux  Inputs=1
      mask Display: e = 0.06;c1 = [120 150 230]/255;c2 = ([120 150 230]+0)/383;c3 = ([120 150 230]+128)/383;patch([0 1 1 0],[0 0 1 1],c1);patch([0 1 1 1-e 1-e 0+e],[0 0 1 1-e 0+e 0+e],c2);patch([0 0 1 1-e 0+e 0+e],[0 1 1 1-e 1-e 0+e],c3);plot([0 1 1 0 0],[0 0 1 1 0]);disp('Mux')
  "pd{2,1}" : Outport
      mask Display: e = 0.06;c1 = [120 230 180]/255;c2 = ([120 230 180]+0)/(256+128);c3 = ([120 230 180]+128)/(256+128);patch([0 1 1 0],[0 0 1 1],c1);patch([0 1 1 1-e 1-e 0+e],[0 0 1 1-e 0+e 0+e],c2);patch([0 0 1 1-e 0+e 0+e],[0 1 1 1-e 1-e 0+e],c3);plot([0 1 1 0 0],[0 0 1 1 0]);
  wires:
  "p{2}"/1 -> mux/1
  mux/1 -> "pd{2,1}"/1

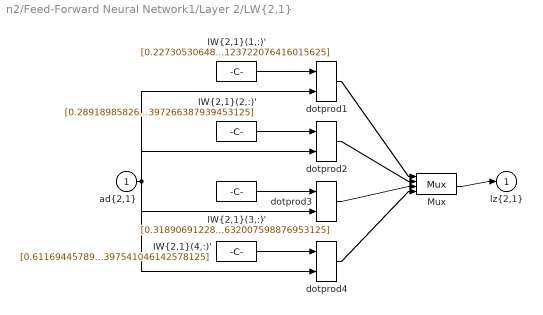
== system n2/Feed-Forward Neural Network1/Layer 2/LW{2,1} ==
  "ad{2,1}" : Inport  PortDimensions=45
      mask Display: e = 0.06;c1 = [120 230 180]/255;c2 = ([120 230 180]+0)/(256+128);c3 = ([120 230 180]+128)/(256+128);patch([0 1 1 0],[0 0 1 1],c1);patch([0 1 1 1-e 1-e 0+e],[0 0 1 1-e 0+e 0+e],c2);patch([0 0 1 1-e 0+e 0+e],[0 1 1 1-e 1-e 0+e],c3);plot([0 1 1 0 0],[0 0 1 1 0]);
  "IW{2,1}(1,:)'" : Constant  Value=[0.2273053064856317140307595536796725355088710784912109375;1.051125980489695077579881399287842214107513427734375;1.204732185290700474666891750530339777469635009765625;-0.025018572614739810477946235778290429152548313140869140625;-0.00749627314337295534707461541756856604479253292083740234375;-0.5694412335341618724982026833458803594112396240234375;0.675417918652810644886130830855108797550201416015625;-0.041349176122834237212533281535797868855297565460205078125;-0.2982536190977691514802927486016415059566497802734375;1.9506673324297765237389512549270875751972198486328125;0.94946659768488850250633959149126894772052764892578125;-0.321528705123451941094714356950134970247745513916015625;1.354552050976334243159726611338555812835693359375;-0.77122036352297096417629518327885307371616363525390625;2.590085879406006430514253224828280508518218994140625;-0.9571395872409185212603688341914676129817962646484375;1.0849524824139880063711416369187645614147186279296875;0.80928673998949707257821728489943780004978179931640625;0.4268521105938030135718008750700391829013824462890625;-0.1996045918910523131462042556449887342751026153564453125;-1.001589388233792732307847472839057445526123046875;-2.26378840025767491539454567828215658664703369140625;1.0241719726556564040720331831835210323333740234375;1.0145500756415994914050315856002271175384521484375;1.0657290722379884062576138603617437183856964111328125;1.29415753393445687180474124033935368061065673828125;0.2468926553676046020679990533608361147344112396240234375;1.780489203995555325121813439182005822658538818359375;0.6167064771087213959077644176431931555271148681640625;-0.446467053105240319066382426171912811696529388427734375;1.5100205275863276543901747572817839682102203369140625;0.61340678180915830797204080226947553455829620361328125;-0.74423736604692869445187852761591784656047821044921875;-1.3211550709702029049452676190412603318691253662109375;-0.2398430918639109510337448227801360189914703369140625;-0.1489453456032401590380942479896475560963153839111328125;-0.85485444250689190948122586632962338626384735107421875;-0.295903939737882371030508465992170386016368865966796875;0.304738340729954371166599003117880783975124359130859375;1.62039485512379233256297084153629839420318603515625;0.1372061016330217431136162531402078457176685333251953125;-0.84434986889209950877699384363950230181217193603515625;-1.4296327550238270287508157707634381949901580810546875;0.99070382423057079535055891028605401515960693359375;-0.253331895238499582578839408597559668123722076416015625]
      mask Display: e = 0.06;c1 = [120 150 230]/255;c2 = ([120 150 230]+0)/383;c3 = ([120 150 230]+128)/383;patch([0 1 1 0],[0 0 1 1],c1);patch([0 1 1 1-e 1-e 0+e],[0 0 1 1-e 0+e 0+e],c2);patch([0 0 1 1-e 0+e 0+e],[0 1 1 1-e 1-e 0+e],c3);plot([0 1 1 0 0],[0 0 1 1 0]);disp('weights');
  "IW{2,1}(2,:)'" : Constant  Value=[0.289189858267777155642619391073822043836116790771484375;1.908173959396009866651411357452161610126495361328125;-0.44814312342037265768368570206803269684314727783203125;-0.33988441742216235486040432078880257904529571533203125;0.44428445852824205442033189683570526540279388427734375;0.01841712340100175315793507024864084087312221527099609375;1.321884955121377824838191372691653668880462646484375;0.5987954868767577654153910771128721535205841064453125;-0.8884258236918942674975596673903055489063262939453125;0.68168303243944539104859359213151037693023681640625;0.01241457478729902051683975372498025535605847835540771484375;0.095605829710638356999652387457899749279022216796875;-0.92839896384661724226816659211181104183197021484375;0.4194250381323045839820906621753238141536712646484375;-0.4000819699081945568508444921462796628475189208984375;1.54065839786964620117259983089752495288848876953125;0.068143673400450632815505969119840301573276519775390625;-0.34966967194239340077643873883062042295932769775390625;-0.1990874832375168768106021843777853064239025115966796875;-1.6613633543110619683602635632269084453582763671875;0.270629138753107734149949692437076009809970855712890625;-6.82876497003395410700932188774459064006805419921875;0.61155811799179160548334266422898508608341217041015625;1.8249679707152370866651835967786610126495361328125;-0.87377775562937032294286154865403659641742706298828125;-0.049080645672161728187976592607810744084417819976806640625;-0.265677825844765624907495293882675468921661376953125;-1.427382742372170110201068382593803107738494873046875;1.1155394234324631508314951133797876536846160888671875;-2.448948341701968178796278152731247246265411376953125;1.4709645068086363295378760085441172122955322265625;-0.2143972810662315431340374516366864554584026336669921875;0.8476818667661636386156942535308189690113067626953125;-1.28025779809898754280084176571108400821685791015625;-0.1530687634671590580115463353649829514324665069580078125;1.2574358444671454027030677025322802364826202392578125;-0.192342401398041484839041004306636750698089599609375;-1.1475468192302524794712326183798722922801971435546875;-0.60210863741174325269867040333338081836700439453125;0.66137222552369545613970558406435884535312652587890625;0.33807858089662878864345429974491707980632781982421875;-0.77278716796796176335959671632735989987850189208984375;-1.3484551884796751597406228029285557568073272705078125;0.256512918706915893363174063779297284781932830810546875;0.69519614536082674494110733576235361397266387939453125]
      mask Display: e = 0.06;c1 = [120 150 230]/255;c2 = ([120 150 230]+0)/383;c3 = ([120 150 230]+128)/383;patch([0 1 1 0],[0 0 1 1],c1);patch([0 1 1 1-e 1-e 0+e],[0 0 1 1-e 0+e 0+e],c2);patch([0 0 1 1-e 0+e 0+e],[0 1 1 1-e 1-e 0+e],c3);plot([0 1 1 0 0],[0 0 1 1 0]);disp('weights');
  "IW{2,1}(3,:)'" : Constant  Value=[0.318906912280309040585990487670642323791980743408203125;-0.4473631263362047860709935775958001613616943359375;0.38862506300972288197925763597595505416393280029296875;-0.212637407641679099246090345332049764692783355712890625;-1.1609584361917628658744661152013577520847320556640625;0.960143937663552993200255514238961040973663330078125;-0.08321205095428797771095474899993860162794589996337890625;-0.55503667882106821895860093718511052429676055908203125;0.189702590396835846231482491930364631116390228271484375;-0.348009796707237029078640944135258905589580535888671875;-1.2740561752481287527416498051024973392486572265625;0.297334546863168680541633648317656479775905609130859375;-1.9706602276936597828438380020088516175746917724609375;0.06452287265000046512231079987031989730894565582275390625;-0.685365605523443388591431357781402766704559326171875;1.3749724961680644952366492361761629581451416015625;-1.3749922377460628286627297711675055325031280517578125;-1.151410498563971263052962967776693403720855712890625;-0.5279967197549237933884569429210387170314788818359375;0.378238456077931550769477553330943919718265533447265625;1.07592211467709564232109187287278473377227783203125;2.528304933603002790931668641860596835613250732421875;-0.9916895721507315020204487154842354357242584228515625;-1.2815125672374261256436511757783591747283935546875;-1.0716190736817974293870747715118341147899627685546875;-0.98626631776197282164275748073123395442962646484375;-0.2880896734473650244723330615670420229434967041015625;-0.80360843469583775888764876071945764124393463134765625;-0.83690443932585456554562597375479526817798614501953125;0.69082708193472119884148696655756793916225433349609375;-0.422012341039969818279331548183108679950237274169921875;-0.461026367428885197607968393640476278960704803466796875;0.83746515456205228300490261972299776971340179443359375;1.1677232298711544000724416036973707377910614013671875;0.3906304139872902592145464950590394437313079833984375;0.1409487274894629660337841414730064570903778076171875;0.25789051861260425813071606171433813869953155517578125;0.423943670453651166862840682370006106793880462646484375;0.2820905381242642118166941145318560302257537841796875;-0.7876438618155301440992843708954751491546630859375;-0.55186288484196255321734270182787440717220306396484375;0.74972528924094949953627065042383037507534027099609375;2.0283777846997654847882586182095110416412353515625;0.59613348555874268175358565713395364582538604736328125;-0.1922916087871342771808969018820789642632007598876953125]
      mask Display: e = 0.06;c1 = [120 150 230]/255;c2 = ([120 150 230]+0)/383;c3 = ([120 150 230]+128)/383;patch([0 1 1 0],[0 0 1 1],c1);patch([0 1 1 1-e 1-e 0+e],[0 0 1 1-e 0+e 0+e],c2);patch([0 0 1 1-e 0+e 0+e],[0 1 1 1-e 1-e 0+e],c3);plot([0 1 1 0 0],[0 0 1 1 0]);disp('weights');
  "IW{2,1}(4,:)'" : Constant  Value=[0.6116944578958187772599330855882726609706878662109375;0.546790257442375970953207797720097005367279052734375;-1.199538468039558214428552673780359327793121337890625;-0.868485284702682935886741688591428101062774658203125;-1.0764968839797186550555352368974126875400543212890625;-0.960256331603024815279923132038675248622894287109375;2.261189207553360613900395037489943206310272216796875;0.380765087269307078710056657655513845384120941162109375;0.42954283533080561685579823461011983454227447509765625;-1.07204086335429504828198332688771188259124755859375;2.84553619137759294943634813535027205944061279296875;-1.627678152868060390545679183560423552989959716796875;0.0816699330526421130027614481150521896779537200927734375;0.9524392060951425431625239070854149758815765380859375;0.29709775055751463934683442857931368052959442138671875;-4.122733803434289967526638065464794635772705078125;1.417712726824593705288179990020580589771270751953125;-1.945068403205659546273409432615153491497039794921875;1.4128882817278187733478489462868310511112213134765625;2.108344024366892721644717312301509082317352294921875;-2.653759788329306701371024246327579021453857421875;7.43098390541018005706064286641776561737060546875;1.4645953713267061413461078700493089854717254638671875;0.7394724307826674447596815298311412334442138671875;-2.16911715681872241390237832092680037021636962890625;0.370990635772849908224912951482110656797885894775390625;0.69844004318589159030494784019538201391696929931640625;2.071414876955594674967642276897095143795013427734375;0.67835372857702169735460984156816266477108001708984375;-1.4990018864692127298354762388044036924839019775390625;0.1380656477586529595757980359849170781672000885009765625;-0.8468277544726252603624061521259136497974395751953125;-0.7915663583833942862355570468935184180736541748046875;-0.037110023873141613492965262821599026210606098175048828125;1.5619033047722241658306074896245263516902923583984375;-2.455826754715367155057492709602229297161102294921875;0.69044711907954614549254301891778595745563507080078125;0.491762755691768471688618546977522782981395721435546875;0.04650543626607621383595159159085596911609172821044921875;0.062153364971660067517245096269107307307422161102294921875;-0.5139023709222370062121854061842896044254302978515625;0.52744162195861343800373788326396606862545013427734375;0.81683286992977011120586894321604631841182708740234375;-0.006007358779311917050536262507876017480157315731048583984375;-0.268857191087297942022615870882873423397541046142578125]
      mask Display: e = 0.06;c1 = [120 150 230]/255;c2 = ([120 150 230]+0)/383;c3 = ([120 150 230]+128)/383;patch([0 1 1 0],[0 0 1 1],c1);patch([0 1 1 1-e 1-e 0+e],[0 0 1 1-e 0+e 0+e],c2);patch([0 0 1 1-e 0+e 0+e],[0 1 1 1-e 1-e 0+e],c3);plot([0 1 1 0 0],[0 0 1 1 0]);disp('weights');
  Mux : Mux
      mask Display: e = 0.06;c1 = [120 150 230]/255;c2 = ([120 150 230]+0)/383;c3 = ([120 150 230]+128)/383;patch([0 1 1 0],[0 0 1 1],c1);patch([0 1 1 1-e 1-e 0+e],[0 0 1 1-e 0+e 0+e],c2);patch([0 0 1 1-e 0+e 0+e],[0 1 1 1-e 1-e 0+e],c3);plot([0 1 1 0 0],[0 0 1 1 0]);disp('Mux');
  dotprod{1..4} (4 alike) : neural/Weight Functions/dotprod
  "lz{2,1}" : Outport
      mask Display: e = 0.06;c1 = [120 230 180]/255;c2 = ([120 230 180]+0)/(256+128);c3 = ([120 230 180]+128)/(256+128);patch([0 1 1 0],[0 0 1 1],c1);patch([0 1 1 1-e 1-e 0+e],[0 0 1 1-e 0+e 0+e],c2);patch([0 0 1 1-e 0+e 0+e],[0 1 1 1-e 1-e 0+e],c3);plot([0 1 1 0 0],[0 0 1 1 0]);
  wires:
  "IW{2,1}(1,:)'"/1 -> dotprod1/1
  "ad{2,1}"/1 -> dotprod1/2, dotprod2/2, dotprod3/2, dotprod4/2
  dotprod1/1 -> Mux/1
  "IW{2,1}(2,:)'"/1 -> dotprod2/1
  dotprod2/1 -> Mux/2
  "IW{2,1}(3,:)'"/1 -> dotprod3/1
  dotprod3/1 -> Mux/3
  "IW{2,1}(4,:)'"/1 -> dotprod4/1
  dotprod4/1 -> Mux/4
  Mux/1 -> "lz{2,1}"/1

== system n2/Feed-Forward Neural Network1/Layer 3/Delays 1 ==
  "p{3}" : Inport  PortDimensions=4
      mask Display: e = 0.06;c1 = [120 230 180]/255;c2 = ([120 230 180]+0)/(256+128);c3 = ([120 230 180]+128)/(256+128);patch([0 1 1 0],[0 0 1 1],c1);patch([0 1 1 1-e 1-e 0+e],[0 0 1 1-e 0+e 0+e],c2);patch([0 0 1 1-e 0+e 0+e],[0 1 1 1-e 1-e 0+e],c3);plot([0 1 1 0 0],[0 0 1 1 0]);
  mux : Mux  Inputs=1
      mask Display: e = 0.06;c1 = [120 150 230]/255;c2 = ([120 150 230]+0)/383;c3 = ([120 150 230]+128)/383;patch([0 1 1 0],[0 0 1 1],c1);patch([0 1 1 1-e 1-e 0+e],[0 0 1 1-e 0+e 0+e],c2);patch([0 0 1 1-e 0+e 0+e],[0 1 1 1-e 1-e 0+e],c3);plot([0 1 1 0 0],[0 0 1 1 0]);disp('Mux')
  "pd{3,2}" : Outport
      mask Display: e = 0.06;c1 = [120 230 180]/255;c2 = ([120 230 180]+0)/(256+128);c3 = ([120 230 180]+128)/(256+128);patch([0 1 1 0],[0 0 1 1],c1);patch([0 1 1 1-e 1-e 0+e],[0 0 1 1-e 0+e 0+e],c2);patch([0 0 1 1-e 0+e 0+e],[0 1 1 1-e 1-e 0+e],c3);plot([0 1 1 0 0],[0 0 1 1 0]);
  wires:
  "p{3}"/1 -> mux/1
  mux/1 -> "pd{3,2}"/1
